simulink model "test_mode0"  (R2024b)
settings: Solver=FixedStepAuto  StartTime=0.0  StopTime=10.0  RelTol=1e-3
settings Model: Creator=rcmas  LastModifiedBy=ben
settings OptimizationCC: DefaultParameterBehavior=Inlined  EnhancedBackFolding=on  PassReuseOutputArgsAs=Individual arguments  ZeroExternalMemoryAtStartup=off  ZeroInternalMemoryAtStartup=off  OptimizeBlockOrder=speed  DifferentSizesBufferReuse=on  OptimizationCustomize=off  EfficientTunableParamExpr=on
settings DebuggingCC: ParameterTunabilityLossMsg=error
settings HardwareCC: ProdBitPerPointer=32  ProdBitPerSizeT=32  ProdBitPerPtrDiffT=32  ProdLargestAtomicInteger=Long  ProdLargestAtomicFloat=Double  ProdWordSize=32  ProdHWDeviceType=ARM Compatible->ARM Cortex-M
settings SFSimCC: MATLABDynamicMemAlloc=off
settings RTWCC: Description=Embedded Coder  SystemTargetFile=ert.tlc  GenCodeOnly=on  PackageGeneratedCodeAndArtifacts=on  TemplateMakefile=ert_default_tmf  Toolchain=GNU gcc/g++ | gmake (64-bit Linux)  TargetLang=C++  HalideCodeGeneration=on
settings CodeAppCC: ForceParamTrailComments=on  IgnoreCustomStorageClasses=off  OperatorAnnotations=on  SimulinkDataObjDesc=on  SFDataObjDesc=on  InsertBlockDesc=on
settings ERTTargetCC: TargetLangStandard=C++17 (ISO)  CodeInterfacePackaging=C++ class  RootIOFormat=Structure reference  ERTCustomFileTemplate=example_file_process.tlc  ArrayContainerType=std::array

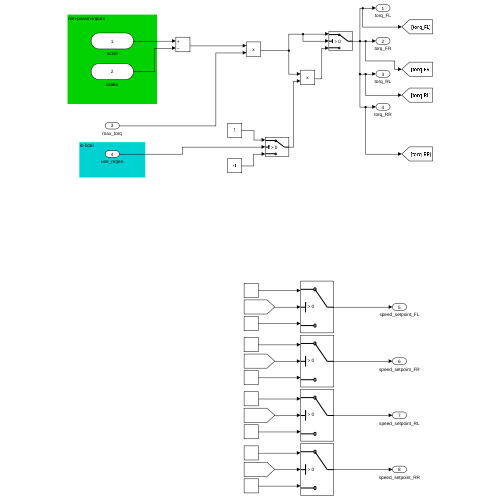
[thumbnail: Simulink's stored preview of the top-level diagram]
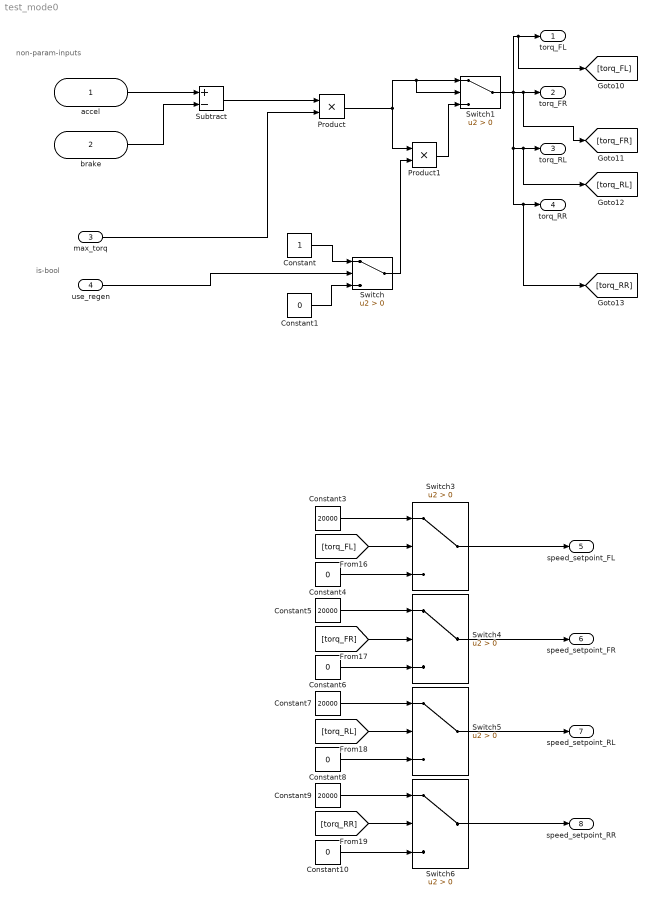
== system test_mode0 ==
  note: non-param-inputs
  note: is-bool
  accel : Inport
  brake : Inport  Port=2
  max_torq : Inport  Port=3
  use_regen : Inport  Port=4
  Constant : Constant
  Constant{1,4,6,8,10} (5 alike) : Constant  Value=0
  Constant{3,5,7,9} (4 alike) : Constant  Value=20000
  Product : Product
  Product1 : Product
  Subtract : Sum  Inputs=+-
  Switch{,1,3..6} (6 alike) : Switch  Criteria=u2 > Threshold  SaturateOnIntegerOverflow=off  InputSameDT=off
  torq_FL : Outport
  torq_FR : Outport  Port=2
  torq_RL : Outport  Port=3
  torq_RR : Outport  Port=4
  speed_setpoint_FL : Outport  Port=5
  speed_setpoint_FR : Outport  Port=6
  speed_setpoint_RL : Outport  Port=7
  speed_setpoint_RR : Outport  Port=8
  wires:
  max_torq/1 -> Product/2
  accel/1 -> Subtract/1
  brake/1 -> Subtract/2
  Subtract/1 -> Product/1
  use_regen/1 -> Switch/2
  Product/1 -> Product1/1, Switch1/2, Switch1/1
  Constant/1 -> Switch/1
  Constant1/1 -> Switch/3
  Switch/1 -> Product1/2
  Product1/1 -> Switch1/3
  Switch1/1 -> [torq_FR], torq_FR/1, [torq_FL], torq_FL/1, [torq_RR], torq_RR/1, [torq_RL], torq_RL/1
  Constant4/1 -> Switch3/3
  Switch6/1 -> speed_setpoint_RR/1
  Switch3/1 -> speed_setpoint_FL/1
  Constant9/1 -> Switch6/1
  Constant7/1 -> Switch5/1
  [torq_RR] -> Switch6/2
  Constant3/1 -> Switch3/1
  Constant10/1 -> Switch6/3
  Switch5/1 -> speed_setpoint_RL/1
  Constant8/1 -> Switch5/3
  [torq_RL] -> Switch5/2
  [torq_FR] -> Switch4/2
  Constant6/1 -> Switch4/3
  Switch4/1 -> speed_setpoint_FR/1
  [torq_FL] -> Switch3/2
  Constant5/1 -> Switch4/1
